simulink model "Practica5_ObservadorLazoCerrado"  (R2022a)
settings: Solver=ode4  StartTime=0.0  StopTime=15  FixedStep=0.001  RelTol=1e-3
model workspace (MAT data in the model file):
  ci = 5
settings Model: Creator=edgar  LastModifiedBy=Anahi Monserrat
settings ModelReferenceCC: EnableRefExpFcnMdlSchedulingChecks=off
settings RTWCC: Description=Generic Real-Time Target

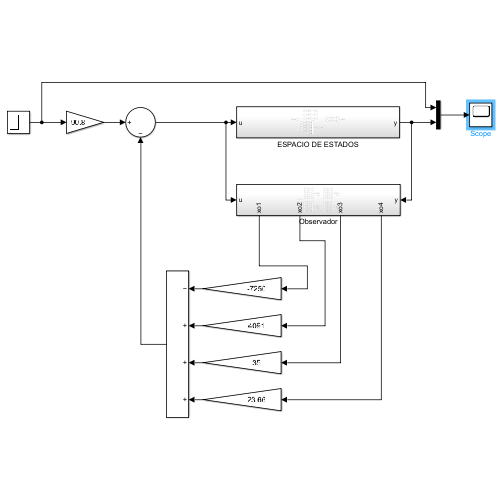
[thumbnail: Simulink's stored preview of the top-level diagram]
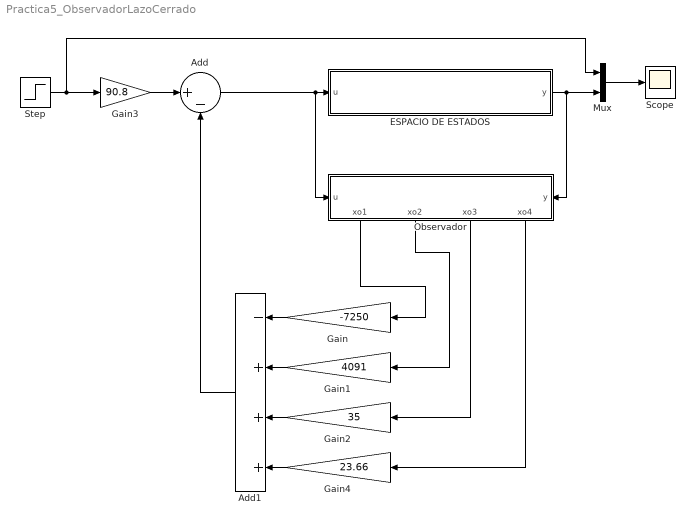
== system Practica5_ObservadorLazoCerrado ==
  Add : Sum  Inputs=|+-
  Add1 : Sum  Inputs=-+++
  ESPACIO DE ESTADOS : Subsystem
  Gain : Gain  Gain=-7250
  Gain1 : Gain  Gain=4091
  Gain2 : Gain  Gain=35
  Gain3 : Gain  Gain=90.8
  Gain4 : Gain  Gain=23.66
  Mux : Mux  Inputs=2
  Observador : Subsystem
      settings: PortSchema="{\"entries\":[{\"content\":{\"sides\":[{\"content\":{\"connectorIds\":[\"In1\"]},\"type\":\"ConnectorPlacement.EquallySpacedRectSide\",\"uuid\":\"cad0d0da-4eac-49d4-839f-d9239b557f86\"},{\"content\":{\"connectorIds\":[\"In2\"],\"side\":\"RIGHT\"},\"type\":\"ConnectorPlacement.EquallySpacedRectSide\",\"uuid\":\"de9e284f-829b-40d7-81eb-b3dcf3e7345e\"},{\"content\":{\"connectorIds\":[],\"side\":\"TOP\"},\"type\":\"ConnectorPlacement.EquallySpacedRectSide\",\"uuid\":\"fab4216e-954a-4506-86c7-96b29bc00207\"},{\"content\":{\"connectorIds\":[\"Out1\",\"Out2\",\"Out3\",\"Out4\"],\"side\":\"BOTTOM\"},\"type\":\"ConnectorPlacement.EquallySpacedRectSide\",\"uuid\":\"cc8ef685-9fff-4377-b971-31d28dc1b4e3\"}]},\"type\":\"ConnectorPlacement.EquallySpacedConnector\",\"uuid\":\"664dda9e-f5b1-4bd1-9822-3917e362ccff\"}],\"packageUris\":[\"http://schema.mathworks.com/mf0/Connector/R2020b\"],\"version\":\"1.0\"}"
  Scope : Scope
  Step : Step  SampleTime=0
  wires:
  Gain3/1 -> Add/1
  Gain1/1 -> Add1/2
  ESPACIO DE ESTADOS/1(y) -> Observador/2(y), Mux/2
  Gain2/1 -> Add1/3
  Mux/1 -> Scope/1
  Gain4/1 -> Add1/4
  Add1/1 -> Add/2
  Step/1 -> Mux/1, Gain3/1
  Gain/1 -> Add1/1
  Add/1 -> Observador/1(u), ESPACIO DE ESTADOS/1(u)
  Observador/1(xo1) -> Gain/1
  Observador/2(xo2) -> Gain1/1
  Observador/3(xo3) -> Gain2/1
  Observador/4(xo4) -> Gain4/1

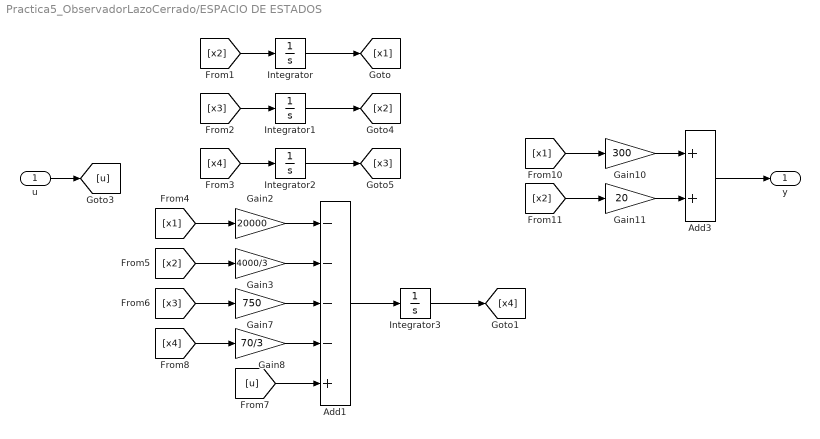
== system Practica5_ObservadorLazoCerrado/ESPACIO DE ESTADOS ==
  u : Inport
  Add1 : Sum  Inputs=----+
  Add3 : Sum
  Gain10 : Gain  Gain=300
  Gain11 : Gain  Gain=20
  Gain2 : Gain  Gain=20000
  Gain3 : Gain  Gain=4000/3
  Gain7 : Gain  Gain=750
  Gain8 : Gain  Gain=70/3
  Integrator{,1..3} (4 alike) : Integrator
  y : Outport
  wires:
  [x1] -> Gain10/1
  Gain10/1 -> Add3/1
  Gain11/1 -> Add3/2
  u/1 -> [u]
  [x2] -> Gain11/1
  Add3/1 -> y/1
  [x4] -> Integrator2/1
  [x3] -> Integrator1/1
  Integrator/1 -> [x1]
  [x2] -> Integrator/1
  Add1/1 -> Integrator3/1
  Integrator3/1 -> [x4]
  [x2] -> Gain3/1
  [x1] -> Gain2/1
  Gain3/1 -> Add1/2
  [x4] -> Gain8/1
  Gain8/1 -> Add1/4
  [u] -> Add1/5
  Integrator1/1 -> [x2]
  [x3] -> Gain7/1
  Gain2/1 -> Add1/1
  Gain7/1 -> Add1/3
  Integrator2/1 -> [x3]

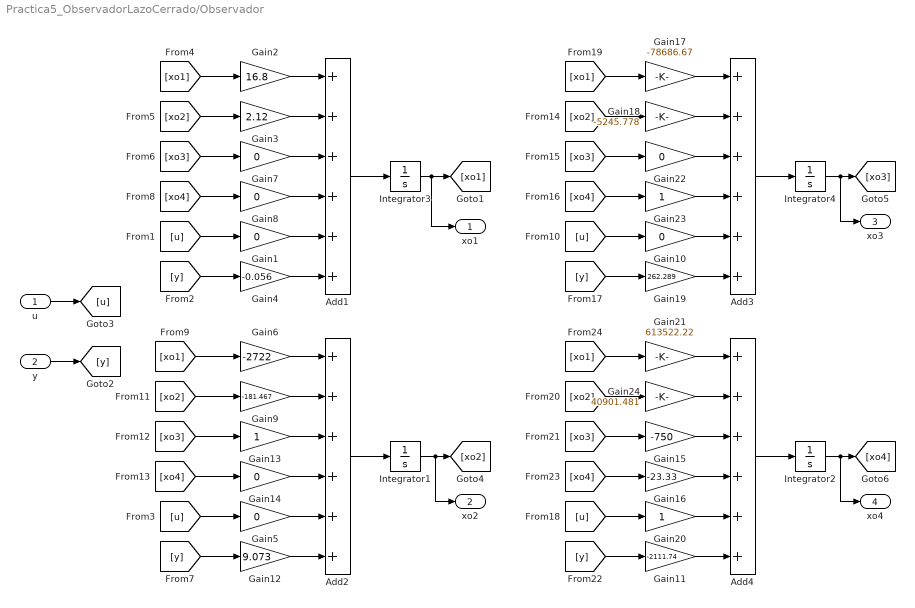
== system Practica5_ObservadorLazoCerrado/Observador ==
  u : Inport
  y : Inport  Port=2
  Add{1..4} (4 alike) : Sum  Inputs=++++++
  Gain{1,5,7..8,10,14,22} (7 alike) : Gain  Gain=0
  Gain11 : Gain  Gain=-2111.74
  Gain12 : Gain  Gain=9.073
  Gain13 : Gain
  Gain15 : Gain  Gain=-750
  Gain16 : Gain  Gain=-23.33
  Gain17 : Gain  Gain=-78686.67
  Gain18 : Gain  Gain=-5245.778
  Gain19 : Gain  Gain=262.289
  Gain2 : Gain  Gain=16.8
  Gain20 : Gain
  Gain21 : Gain  Gain=613522.22
  Gain23 : Gain
  Gain24 : Gain  Gain=40901.481
  Gain3 : Gain  Gain=2.12
  Gain4 : Gain  Gain=-0.056
  Gain6 : Gain  Gain=-2722
  Gain9 : Gain  Gain=-181.467
  Integrator{1..4} (4 alike) : Integrator
  xo1 : Outport
  xo2 : Outport  Port=2
  xo3 : Outport  Port=3
  xo4 : Outport  Port=4
  wires:
  Gain7/1 -> Add1/3
  Gain2/1 -> Add1/1
  [xo3] -> Gain7/1
  Gain8/1 -> Add1/4
  [xo4] -> Gain8/1
  Gain3/1 -> Add1/2
  [xo1] -> Gain2/1
  [xo2] -> Gain3/1
  Integrator3/1 -> xo1/1, [xo1]
  Add1/1 -> Integrator3/1
  u/1 -> [u]
  y/1 -> [y]
  [y] -> Gain4/1
  [u] -> Gain1/1
  Gain1/1 -> Add1/5
  Gain4/1 -> Add1/6
  Gain12/1 -> Add2/6
  Gain5/1 -> Add2/5
  [u] -> Gain5/1
  [y] -> Gain12/1
  Add2/1 -> Integrator1/1
  Integrator1/1 -> xo2/1, [xo2]
  [xo2] -> Gain9/1
  [xo1] -> Gain6/1
  Gain9/1 -> Add2/2
  [xo4] -> Gain14/1
  Gain14/1 -> Add2/4
  [xo3] -> Gain13/1
  Gain6/1 -> Add2/1
  Gain13/1 -> Add2/3
  Gain15/1 -> Add4/3
  Gain21/1 -> Add4/1
  [xo3] -> Gain15/1
  Gain16/1 -> Add4/4
  [xo4] -> Gain16/1
  Gain24/1 -> Add4/2
  [xo1] -> Gain21/1
  [xo2] -> Gain24/1
  Integrator2/1 -> xo4/1, [xo4]
  Add4/1 -> Integrator2/1
  [y] -> Gain11/1
  [u] -> Gain20/1
  Gain20/1 -> Add4/5
  Gain11/1 -> Add4/6
  Gain19/1 -> Add3/6
  Gain10/1 -> Add3/5
  [u] -> Gain10/1
  [y] -> Gain19/1
  Add3/1 -> Integrator4/1
  Integrator4/1 -> xo3/1, [xo3]
  [xo2] -> Gain18/1
  [xo1] -> Gain17/1
  Gain18/1 -> Add3/2
  [xo4] -> Gain23/1
  Gain23/1 -> Add3/4
  [xo3] -> Gain22/1
  Gain17/1 -> Add3/1
  Gain22/1 -> Add3/3
